simulink model "Copy_of_test_controler_int"  (R2015a)
settings: Solver=FixedStepDiscrete  StartTime=0.0  StopTime=30  RelTol=1e-3
values from neighbouring files (symbols this model uses):
  K = dlqr(A, B, Q, R)    [teste_integrador.m]
  M = dlqe(A, G, C, Qw, Rw)    [teste_integrador.m]
  Nbar = Nu+K*Nx    [teste_integrador.m]
undefined symbols (not defined in the file or in its folder): A, B, C, T
settings Model: Creator=alunos  LastModifiedBy=alunos
settings DataIOCC: LimitDataPoints=off

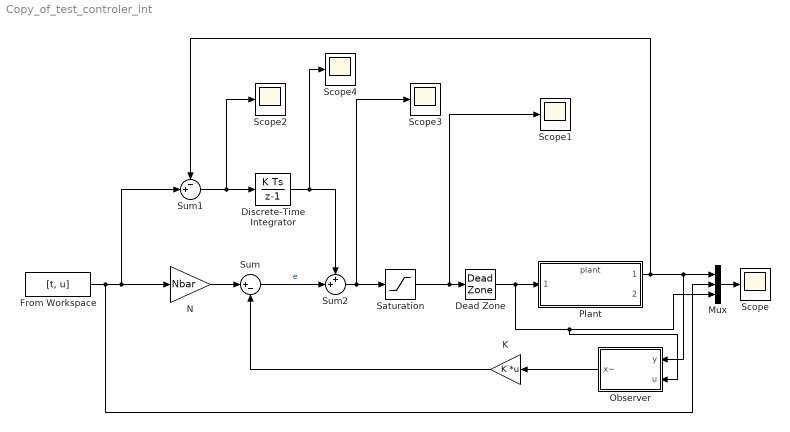
== system Copy_of_test_controler_int ==
  Dead Zone : DeadZone  LowerValue=-0.28  UpperValue=0.3  SaturateOnIntegerOverflow=on
  Discrete-Time Integrator : DiscreteIntegrator  gainval=Ki  InitialConditionSetting=State (most efficient)  SampleTime=-1
  From Workspace : FromWorkspace  VariableName=[t, u]  SampleTime=T
  K : Gain  Gain=K  Multiplication=Matrix(K*u)
  Mux : Mux  Inputs=3
  N : Gain  Gain=Nbar
  Observer : Subsystem
  Plant : ModelReference  ModelNameDialog=plant.slx  SimulationMode=Normal  ModelReferenceVersion=1.9  CopyOfModelName=plant.slx  DefaultDataLogging=on
  Saturation : Saturate  UpperLimit=10  LowerLimit=-10
  Scope{,1..4} (5 alike) : Scope
      Scope settings: SaveName=test_controller
      Scope1 settings: SaveName=test_controller1
      Scope2 settings: SaveName=test_controller2
      Scope3 settings: SaveName=test_controller3
      Scope4 settings: SaveName=test_controller4
  Sum : Sum  Inputs=|+-
  Sum1 : Sum  Inputs=-+|
  Sum2 : Sum  Inputs=++|
  wires:
  K/1 -> Sum/2
  Plant/1 -> Sum1/1, Observer/1(y), Mux/1
  Mux/1 -> Scope/1
  Saturation/1 -> Scope1/1, Dead Zone/1
  Dead Zone/1 -> Observer/2(u), Mux/3, Plant/1
  Sum1/1 -> Discrete-Time Integrator/1, Scope2/1
  From Workspace/1 -> Sum1/2, N/1, Mux/2
  N/1 -> Sum/1
  Observer/1(x~) -> K/1
  Sum2/1 -> Scope3/1, Saturation/1
  Sum/1 -> Sum2/2  "e"
  Discrete-Time Integrator/1 -> Scope4/1, Sum2/1

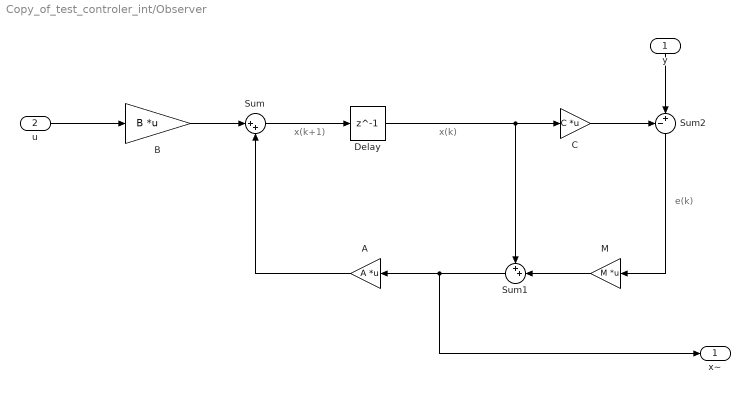
== system Copy_of_test_controler_int/Observer ==
  note: e(k)
  note: x(k)
  note: x(k+1)
  y : Inport  PortDimensions=1
  u : Inport  Port=2
  A : Gain  Gain=A  Multiplication=Matrix(K*u)
  B : Gain  Gain=B  Multiplication=Matrix(K*u) (u vector)
  C : Gain  Gain=C  Multiplication=Matrix(K*u)
  Delay : Delay  DelayLength=1  InitialCondition=[0;0;0;0]
  M : Gain  Gain=M  Multiplication=Matrix(K*u) (u vector)
  Sum : Sum  Inputs=|++
  Sum1 : Sum  Inputs=++|
  Sum2 : Sum  Inputs=-+|
  x~ : Outport  PortDimensions=[4,1]
  wires:
  Sum/1 -> Delay/1
  C/1 -> Sum2/1
  Sum2/1 -> M/1
  Delay/1 -> C/1, Sum1/1
  M/1 -> Sum1/2
  A/1 -> Sum/2
  y/1 -> Sum2/2
  u/1 -> B/1
  Sum1/1 -> x~/1, A/1
  B/1 -> Sum/1
